simulink model "s0303_main"  (R2019b)
settings: Solver=FixedStepAuto  StartTime=0.0  StopTime=T_sim  FixedStep=dt  RelTol=1e-3
undefined symbols (not defined in the file or in its folder): __PRM__SERIALIZED__DATA__, SubsystemReferenceBlock
settings Model: Creator=paolo  LastModifiedBy=giaco
settings DebuggingCC: SFMachineParentedDataDiag=error

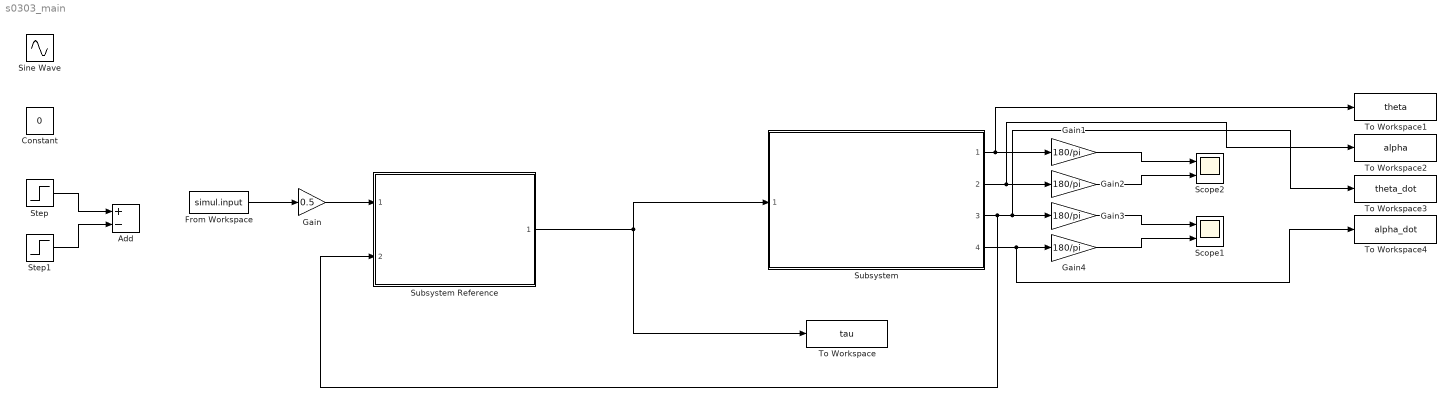
== system s0303_main ==
  Add : Sum  Inputs=+-
  Constant : Constant  Value=0
  From Workspace : FromWorkspace  VariableName=simul.input  SampleTime=0
  Gain : Gain  Gain=0.5
  Gain{1..4} (4 alike) : Gain  Gain=180/pi
  Scope1 : Scope  NumInputPorts=2
  Scope2 : Scope  NumInputPorts=2
  Sine Wave : Sin  Frequency=2*2*pi  SampleTime=0
  Step : Step  SampleTime=0
  Step1 : Step  Time=2  SampleTime=0
  Subsystem : Subsystem  ReferencedSubsystem=s0303_simulator  th_0=0  al_0=0  th_dot_0=0  al_dot_0=0
  Subsystem Reference : Subsystem  BlockKeywords=__PRM__SERIALIZED__DATA__:SubsystemReferenceBlock  ReferencedSubsystem=s0303_motor_simulator  omega_0=0  i_0=0
  To Workspace : ToWorkspace  VariableName=tau  SampleTime=-1
  To Workspace1 : ToWorkspace  VariableName=theta  SampleTime=-1
  To Workspace2 : ToWorkspace  VariableName=alpha  SampleTime=-1
  To Workspace3 : ToWorkspace  VariableName=theta_dot  SampleTime=-1
  To Workspace4 : ToWorkspace  VariableName=alpha_dot  SampleTime=-1
  wires:
  Step/1 -> Add/1
  Step1/1 -> Add/2
  Subsystem/1 -> To Workspace1/1, Gain1/1
  Subsystem/2 -> To Workspace2/1, Gain2/1
  Gain1/1 -> Scope2/1
  Gain2/1 -> Scope2/2
  Subsystem/4 -> To Workspace4/1, Gain4/1
  Gain4/1 -> Scope1/2
  Subsystem/3 -> Subsystem Reference/2, To Workspace3/1, Gain3/1
  Gain3/1 -> Scope1/1
  Subsystem Reference/1 -> Subsystem/1, To Workspace/1
  From Workspace/1 -> Gain/1
  Gain/1 -> Subsystem Reference/1
